simulink model "vbyfcontrolim_interrupt"  (R2016a)
settings: Solver=ode4  StartTime=0.0  StopTime=20  FixedStep=Ts  RelTol=1e-3
values from neighbouring files (symbols this model uses):
  Cdc = 100e-6    (= 0.0001)    [control_simulation_parameters.m]    (also in pmsm_vbyf_sim_parameters.m = 1.5e-05; vbyfcontrolim_sim.m)
  deltad = delta*180/pi    [control_simulation_parameters.m]    (also in pmsm_vbyf_sim_parameters.m)
  Ef = 155    [control_simulation_parameters.m]    (also in pmsm_vbyf_sim_parameters.m = 80)
  fout = 50    [control_simulation_parameters.m]    (also in pmsm_vbyf_sim_parameters.m = 100; vbyfcontrolim_sim.m)
  frated = 50    [vbyfcontrolim_sim.m]
  fsw = 10e3    (= 10000)    [control_simulation_parameters.m]    (also in pmsm_vbyf_sim_parameters.m; vbyfcontrolim_sim.m)
  Ls = 13.8e-3    (= 0.0138)    [control_simulation_parameters.m]
  phase = [0 90 0 90]    [control_simulation_parameters.m]    (also in pmsm_vbyf_sim_parameters.m = [0])
  Rin = 10    [control_simulation_parameters.m]    (also in pmsm_vbyf_sim_parameters.m = 1; vbyfcontrolim_sim.m = 1e-06)
  Ripth = 0.08    [control_simulation_parameters.m]    (also in pmsm_vbyf_sim_parameters.m; vbyfcontrolim_sim.m)
  Rs = 1e-3    (= 0.001)    [control_simulation_parameters.m]
  Tload = 30    [pmsm_vbyf_sim_parameters.m]    (also in vbyfcontrolim_sim.m = 10)
  Trated = Prated/wrated    (= 26.7113191203)    [vbyfcontrolim_sim.m]
  Ts = 100e-9    (= 1e-07)    [control_simulation_parameters.m]    (also in pmsm_vbyf_sim_parameters.m = 1e-06; vbyfcontrolim_sim.m = 1e-06)
  VbyfFreqSteps = 2    [vbyfcontrolim_sim.m]
  VbyfStepTime = 0.2    [vbyfcontrolim_sim.m]
  Vdc = 300    [control_simulation_parameters.m]    (also in pmsm_vbyf_sim_parameters.m = 270; vbyfcontrolim_sim.m = 750)
  Vin = Vdc + Rin*(Pout/Vdc)    (= 366.666666667)    [control_simulation_parameters.m]    (also in pmsm_vbyf_sim_parameters.m = 276.981317008; vbyfcontrolim_sim.m = 750)
  Vrated = Vllrated/sqrt(3)    [vbyfcontrolim_sim.m]
undefined symbols (not defined in the file or in its folder): Initial_freq, Lload, Rload, start_time, start_time_deceleration
libraries: powerlib x25, powerlib_meascontrol x14, simulink x4, dspsigops x2
settings Model: SimulationMode=accelerator  Creator=ugurm  LastModifiedBy=mesutto
settings DataIOCC: LimitDataPoints=on  SaveFormat=Array
settings DebuggingCC: UnderspecifiedInitializationDetection=Classic  MergeDetectMultiDrivingBlocksExec=none  SolverPrmCheckMsg=warning  StateNameClashWarn=warning
settings HardwareCC: ProdBitPerPointer=32  ProdLargestAtomicFloat=None  ProdIntDivRoundTo=Undefined  ProdEndianess=Unspecified  ProdWordSize=32  ProdHWDeviceType=32-bit Generic
settings ModelReferenceCC: PropagateSignalLabelsOutOfModel=off
settings ConfigComp: CovModelRefEnable=Off

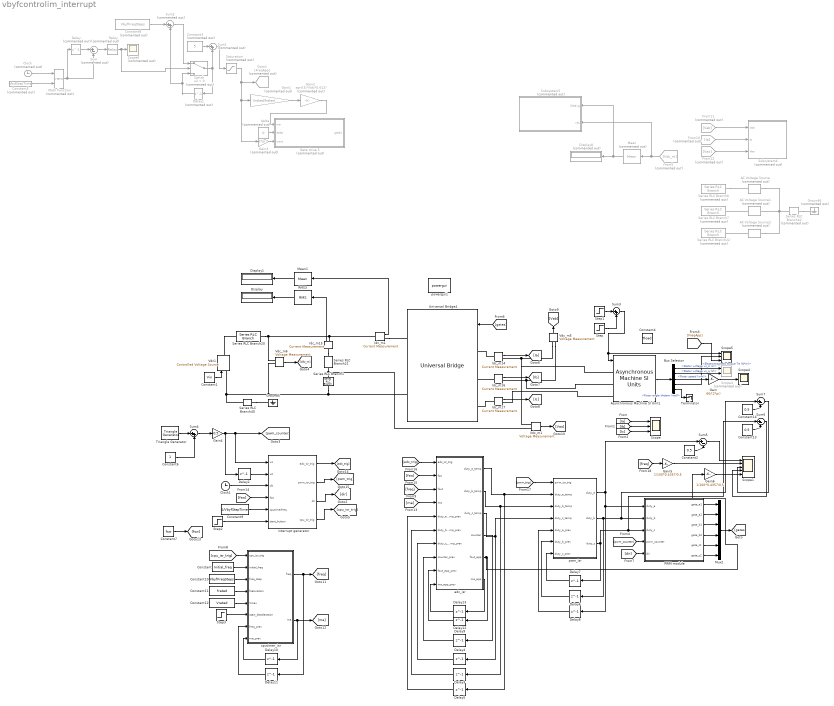
== system vbyfcontrolim_interrupt ==
  AC Voltage Source : powerlib/Electrical Sources/AC Voltage Source  Commented=on  Amplitude=Ef*sqrt(2)  Phase=0  Frequency=fout  SampleTime=0  Measurements=None  BusType=swing  Pref=10e3  Qref=0  Qmin=-inf  Qmax=+inf
  AC Voltage Source1 : powerlib/Electrical Sources/AC Voltage Source  Commented=on  Amplitude=Ef*sqrt(2)  Phase=-120  Frequency=fout  SampleTime=0  Measurements=None  BusType=swing  Pref=10e3  Qref=0  Qmin=-inf  Qmax=+inf
  AC Voltage Source2 : powerlib/Electrical Sources/AC Voltage Source  Commented=on  Amplitude=Ef*sqrt(2)  Phase=-240  Frequency=fout  SampleTime=0  Measurements=None  BusType=swing  Pref=10e3  Qref=0  Qmin=-inf  Qmax=+inf
  Asynchronous Machine SI Units : powerlib/Machines/Asynchronous Machine SI Units  RotorType=Squirrel-cage  PresetModel=No  MechanicalLoad=Torque Tm  ShowDetailedParameters=on  ReferenceFrame=Synchronous  Units=SI  MeasurementBus=off  NominalParameters=[4000 400 50]  Stator=[1.405 0.005839]  Rotor=[1.395 0.005839]  Cage1=[0.4155 0.002066]  Cage2=[0.4168 0.0003495]  Lm=0.1722  Mechanical=[0.0131 0.002985 2]  PolePairs=2  InitialConditions=[1 0 0 0 0 0 0 0]  SimulateSaturation=off  Saturation=[14.03593122, 27.81365428, 53.79336849, 72.68890987, 97.98006896, 148.6815601, 215.7428561, 302.9841135, 428.7778367 ; 230, 322, 414, 460, 506, 552, 598, 644, 690]  LoadFlowParameters=1492000  TsPowergui=0  TsBlock=-1  IterativeModel=Trapezoidal non iterative  IterativeDiscreteModel=Trapezoidal non iterative  Pmec=1.492e+006
  Bus Selector : BusSelector  OutputSignals=Stator measurements.Stator voltage vs_d (V),Stator measurements.Stator voltage vs_q (V),Mechanical.Rotor speed (wm),Mechanical.Electromagnetic torque Te (N*m),Mechanical.Rotor angle thetam (rad)
  Clock : Clock  Commented=on
  Clock1 : Clock
  Constant : Constant  Value=Initial_freq
  Constant1 : Constant  Value=Vin
  Constant10 : Constant  Value=VbyfFreqSteps
  Constant11 : Constant  Value=frated
  Constant12 : Constant  Value=Vrated
  Constant13 : Constant  Value=0.5
  Constant14 : Constant  Value=0.5
  Constant2 : Constant  Value=0.5
  Constant3 : Constant  Commented=on  Value=5
  Constant4 : Constant  Value=Tload
  Constant5 : Constant  Commented=on  Value=VbyfStepTime
  Constant6 : Constant
  Constant7 : Constant  Value=fsw
  Constant8 : Constant  Commented=on  Value=VbyfFreqSteps
  Constant9 : Constant  Value=1/VbyfStepTime
  Delay : Delay  Commented=on  DelayLength=1
  Delay1 : Delay  Commented=on  DelayLength=1
  Delay{2..13} (12 alike) : Delay  DelayLength=1
  Display : Display
  Display1 : Display
  Display8 : Display  Commented=on
  From10 : From  Commented=on  GotoTag=Ia
  From11 : From  Commented=on  GotoTag=Vab
  From12 : From  Commented=on  GotoTag=Vao
  From5 : From  Commented=on  GotoTag=Vdc_m
  Gain : Gain  Gain=60/(2*pi)
  Gain1 : Gain  Commented=on  Gain=Vrated/frated
  Gain2 : Gain  Commented=on  Gain=sqrt(3)/(Vdc*0.612)
  Gain3 : Gain  Commented=on  Gain=2*pi
  Gain4 : Gain  Gain=0.5
  Gain5 : Gain  Gain=1/100*0.4357/0.5
  Gain6 : Gain  Gain=1/100*0.4357/0.5
  Gate drive 5 : Subsystem  Commented=on
  Goto1 : Goto  Commented=on  GotoTag=FreqApp
  Ground5 : powerlib/Elements/Ground  LConnTagsString=a
  Ground6 : powerlib/Elements/Ground  Commented=on  LConnTagsString=a
  Idc_m{1,14..17} (5 alike) : powerlib/Measurements/Current Measurement  PhasorSimulation=off  OutputType=Complex  PSBequivalent=0
  Math Function : Math  Commented=on  Operator=rem  SaturateOnIntegerOverflow=on
  Mean : powerlib_meascontrol/Measurements/Mean  Commented=on  Freq=fout  Vinit=0  Ts=0
  Mean1 : powerlib_meascontrol/Measurements/Mean  Freq=fout  Vinit=0  Ts=0
  Mux2 : Mux  Inputs=6
  PWM module : MATLAB Function  TreatAsAtomicUnit=on
  RMS3 : powerlib_meascontrol/Measurements/RMS  TrueRMS=on  Freq=fout  RMSInit=0  Ts=0
  Relay : Relay  Commented=on
  Saturation : Saturate  Commented=on  UpperLimit=frated  LowerLimit=0
  Scope : Scope  NumInputPorts=3
  Scope1 : Scope  NumInputPorts=5
  Scope3 : Scope  Commented=on  NumInputPorts=2
  Scope4 : Scope
  Scope5 : Scope  NumInputPorts=3
  Scope6 : Scope  Commented=on
  Series RLC Branch1 : powerlib/Elements/Series RLC Branch  LConnTagsString=__new0  RConnTagsString=__new0  BranchType=C  Resistance=Rload  Inductance=Lload  SetiL0=off  InitialCurrent=0  Capacitance=Cdc*2  Setx0=off  InitialVoltage=0  Measurements=None
  Series RLC Branch20 : powerlib/Elements/Series RLC Branch  LConnTagsString=__new0  RConnTagsString=__new0  BranchType=R  Resistance=Rin  Inductance=Lload  SetiL0=off  InitialCurrent=0  Capacitance=1e-6  Setx0=off  InitialVoltage=0  Measurements=None
  Series RLC Branch21 : powerlib/Elements/Series RLC Branch  LConnTagsString=__new0  RConnTagsString=__new0  BranchType=C  Resistance=Rload  Inductance=Lload  SetiL0=off  InitialCurrent=0  Capacitance=Cdc*2  Setx0=off  InitialVoltage=0  Measurements=None
  Series RLC Branch22 : powerlib/Elements/Series RLC Branch  Commented=on  LConnTagsString=__new0  RConnTagsString=__new0  BranchType=RL  Resistance=Rs  Inductance=Ls  SetiL0=off  InitialCurrent=0  Capacitance=1e-6  Setx0=off  InitialVoltage=0  Measurements=None
  Series RLC Branch40 : powerlib/Elements/Series RLC Branch  LConnTagsString=__new0  RConnTagsString=__new0  BranchType=R  Resistance=1e12  Inductance=Lload  SetiL0=off  InitialCurrent=0  Capacitance=1e-6  Setx0=off  InitialVoltage=0  Measurements=None
  Series RLC Branch42 : powerlib/Elements/Series RLC Branch  Commented=on  LConnTagsString=__new0  RConnTagsString=__new0  BranchType=R  Resistance=1e12  Inductance=Lload  SetiL0=off  InitialCurrent=0  Capacitance=1e-6  Setx0=off  InitialVoltage=0  Measurements=None
  Series RLC Branch6 : powerlib/Elements/Series RLC Branch  Commented=on  LConnTagsString=__new0  RConnTagsString=__new0  BranchType=RL  Resistance=Rs  Inductance=Ls  SetiL0=off  InitialCurrent=0  Capacitance=1e-6  Setx0=off  InitialVoltage=0  Measurements=None
  Series RLC Branch7 : powerlib/Elements/Series RLC Branch  Commented=on  LConnTagsString=__new0  RConnTagsString=__new0  BranchType=RL  Resistance=Rs  Inductance=Ls  SetiL0=off  InitialCurrent=0  Capacitance=1e-6  Setx0=off  InitialVoltage=0  Measurements=None
  Step : Step  Time=2  After=Tload  SampleTime=0
  Step1 : Step  Time=6  After=Trated-Tload  SampleTime=0
  Step2 : Step  Time=start_time  SampleTime=0
  Step3 : Step  Time=start_time_deceleration  SampleTime=0
  Subsystem4 : Subsystem  Commented=on
  Subsystem5 : Subsystem  Commented=on
  Sum : Sum  Commented=on  Inputs=|+-
  Sum1 : Sum  Commented=on  Inputs=|++
  Sum2 : Sum  Commented=on  Inputs=|++
  Sum3 : Sum  Inputs=|++
  Sum4 : Sum  Inputs=|++
  Sum5 : Sum  Inputs=|+-
  Sum6 : Sum  Inputs=|+-
  Sum7 : Sum  Inputs=|+-
  Switch : Switch  Commented=on  Criteria=u2 > Threshold
  Terminator : Terminator
  Triangle Generator : powerlib_meascontrol/Pulse & Signal Generators/Triangle Generator  Freq=fsw  Phase=0  Ts=0
  Universal Bridge4 : powerlib/Power Electronics/Universal Bridge  Arms=3  SnubberResistance=1e5  SnubberCapacitance=inf  Device=IGBT / Diodes  Ron=1e-6  Lon=0  ForwardVoltages="[  0  0  ]"  ForwardVoltage=0  GTOparameters=[ 10e-6 , 20e-6 ]  IGBTparameters=[0,0]  Measurements=None  Measurements_2=None  converterType=Rectifier
  Vdc1 : powerlib/Electrical Sources/Controlled Voltage Source  Initialize=off  Source_Type=DC  Amplitude=200  Phase=0  Frequency=0  Measurements=None
  Vdc_m1 : powerlib/Measurements/Voltage Measurement  PhasorSimulation=off  OutputType=Complex  PSBequivalent=0
  Vdc_m5 : powerlib/Measurements/Voltage Measurement  PhasorSimulation=off  OutputType=Complex  PSBequivalent=0
  Vdc_m6 : powerlib/Measurements/Voltage Measurement  PhasorSimulation=off  OutputType=Complex  PSBequivalent=0
  adc_isr : MATLAB Function  TreatAsAtomicUnit=on
  cputimer_isr : MATLAB Function  TreatAsAtomicUnit=on
  delta : Constant  Commented=on  Value=0
  interrupt generator : MATLAB Function  TreatAsAtomicUnit=on
  powergui1 : powerlib/powergui  Priority=1  SimulationMode=Discrete  SolverType=Tustin  SampleTime=Ts  frequency=60  SPID=off  DisableSnubberDevices=off  DisableRonSwitches=off  DisableVfSwitches=off  SwTol=0  DisplayEquations=off  Interpol=off  ExternalGateDelay=off  methode=off  Ts=0  FunctionMessages=off  echomessages=off  HookPort=off  EnableUseOfTLC=off  x0status=blocks  frequencyindice=0  Pbase=100e6  ErrMax=1e-4  Iterations=50  UnitsV=kV  UnitsW=MW  buscounter=0  RestoreLinks=warning  ResistiveCurrentMeasurement=off  Frange=[0:2:500]  Ylog=off  Xlog=on  ShowGrid=off  save=off  variable=ZData  structure=Vdc  ZoomFFT=off  StartTime=0.04  cycles=5  DisplayStyle=5  fundamental=50  FreqAxis=off  MaxFrequency=30000  frequencyindicesteady=1  RmsSteady=1  display=off
  pwm_isr : MATLAB Function  TreatAsAtomicUnit=on
  wires:
  Constant1/1 -> Vdc1/1
  Idc_m15/1 -> RMS3/1
  Vdc_m6/1 -> [Vdc_m]
  RMS3/1 -> Display/1
  Mean/1 -> Subsystem5/1(Vdcavg), Display8/1
  Idc_m1/1 -> Mean1/1
  Mean1/1 -> Display1/1
  Idc_m14/1 -> [Ia]
  From5/1 -> Subsystem5/2(vdc), Mean/1
  From10/1 -> Subsystem4/2(Ia)
  Idc_m16/1 -> [Ib]
  Idc_m17/1 -> [Ic]
  From11/1 -> Subsystem4/1(Vab)
  From12/1 -> Subsystem4/3(Vao)
  Vdc_m5/1 -> [Vab]
  Vdc_m1/1 -> [Vao]
  [Ia] -> Scope/1
  [Ic] -> Scope/3
  [Ib] -> Scope/2
  delta/1 -> Gate drive 5/2(delta)
  Asynchronous Machine SI Units/1 -> Bus Selector/1
  Bus Selector/1 -> Scope3/1  "<Stator voltage vs_d (V)>"
  Bus Selector/2 -> Scope3/2  "<Stator voltage vs_q (V)>"
  Bus Selector/3 -> Gain/1  "<Rotor speed (wm)>"
  Bus Selector/4 -> Scope5/2  "<Electromagnetic torque Te (N*m)>"
  Bus Selector/5 -> Terminator/1  "<Rotor angle thetam (rad)>"
  Gain/1 -> Scope4/1
  Clock/1 -> Math Function/1
  Constant5/1 -> Math Function/2
  Math Function/1 -> Sum/2, Delay/1
  Delay/1 -> Sum/1
  Sum/1 -> Relay/1
  Relay/1 -> Switch/2, Scope6/1
  Sum2/1 -> Switch/1
  Constant8/1 -> Sum2/1
  Delay1/1 -> Switch/3, Sum2/2
  Switch/1 -> Sum1/2, Delay1/1
  Gain1/1 -> Gain2/1
  Gain2/1 -> Gate drive 5/1(ma)
  Gain3/1 -> Gate drive 5/3(wout)
  Saturation/1 -> Goto1/1, Gain3/1, Gain1/1
  Step/1 -> Sum3/2
  [FreqApp] -> Scope5/3
  Constant3/1 -> Sum1/1
  Sum1/1 -> Saturation/1
  Step1/1 -> Sum3/1
  Sum3/1 -> Asynchronous Machine SI Units/1, Scope5/1
  Triangle Generator/1 -> Sum4/1
  Constant6/1 -> Sum4/2
  Sum4/1 -> Gain4/1
  Gain4/1 -> [pwm_counter], interrupt generator/1(u1), Delay2/1
  Delay2/1 -> interrupt generator/2(u2)
  Clock1/1 -> interrupt generator/3(clk)
  adc_isr/1(duty_a_temp) -> Delay5/1, pwm_isr/2(duty_a_temp)
  adc_isr/2(duty_b_temp) -> Delay3/1, pwm_isr/3(duty_b_temp)
  adc_isr/3(duty_c_temp) -> pwm_isr/4(duty_c_temp), Delay4/1
  [pwm_counter] -> PWM module/4(pwm_counter)
  PWM module/6(gate_c2) -> Mux2/6
  PWM module/4(gate_b2) -> Mux2/4
  PWM module/5(gate_c1) -> Mux2/5
  PWM module/3(gate_b1) -> Mux2/3
  PWM module/2(gate_a2) -> Mux2/2
  PWM module/1(gate_a1) -> Mux2/1
  [gates] -> Universal Bridge4/1
  Mux2/1 -> [gates]
  [dir] -> PWM module/5(dir)
  interrupt generator/3(dir) -> [dir]
  Delay5/1 -> adc_isr/5(duty_a_temp_prev)
  Delay3/1 -> adc_isr/6(duty_b_temp_prev)
  Delay4/1 -> adc_isr/7(duty_c_temp_prev)
  Delay7/1 -> pwm_isr/7(duty_c_prev)
  Delay6/1 -> pwm_isr/6(duty_b_prev)
  Delay8/1 -> pwm_isr/5(duty_a_prev)
  pwm_isr/3(duty_c) -> Delay7/1, Sum6/1, PWM module/3(duty_c)
  pwm_isr/1(duty_a) -> Sum5/1, PWM module/1(duty_a), Delay8/1
  [fsw] -> interrupt generator/4(fsw)
  [freq] -> adc_isr/3(fout)
  Delay9/1 -> adc_isr/8(counter_prev)
  Constant9/1 -> interrupt generator/5(cputimerfreq)
  Constant/1 -> cputimer_isr/2(initial_freq)
  interrupt generator/4(cpu_isr_trig) -> [cpu_isr_trig]
  [cpu_isr_trig] -> cputimer_isr/1(cpu_isr_trig)
  Constant10/1 -> cputimer_isr/3(freq_step)
  Constant11/1 -> cputimer_isr/4(fsaturation)
  Constant12/1 -> cputimer_isr/5(Vmax)
  cputimer_isr/2(ma) -> [ma], Delay10/1
  Delay10/1 -> cputimer_isr/8(ma_prev)
  cputimer_isr/1(freq) -> [freq], Delay11/1
  Delay11/1 -> cputimer_isr/7(freq_prev)
  [ma] -> adc_isr/4(ma)
  Constant7/1 -> [fsw]
  [fsw] -> adc_isr/2(fsw)
  interrupt generator/1(adc_isr_trig) -> [adc_trig]
  [adc_trig] -> adc_isr/1(adc_isr_trig)
  interrupt generator/2(pwm_isr_trig) -> [pwm_trig]
  [pwm_trig] -> pwm_isr/1(pwm_isr_trig)
  adc_isr/5(fout_app) -> Gain6/1, Delay12/1
  adc_isr/6(ma_app) -> Delay13/1
  Delay13/1 -> adc_isr/10(ma_app_prev)
  Delay12/1 -> adc_isr/9(fout_app_prev)
  Gain5/1 -> Scope1/2
  [freq] -> Gain5/1
  adc_isr/4(counter) -> Delay9/1
  Constant2/1 -> Sum5/2
  Sum5/1 -> Scope1/1
  Constant13/1 -> Sum6/2
  Constant14/1 -> Sum7/2
  pwm_isr/2(duty_b) -> Sum7/1, PWM module/2(duty_b), Delay6/1
  Sum7/1 -> Scope1/3
  Sum6/1 -> Scope1/4
  Gain6/1 -> Scope1/5
  Step2/1 -> interrupt generator/6(start_button)
  Step3/1 -> cputimer_isr/6(start_deceleration)
  connections:
  Vdc_m5/LConn1 -- Asynchronous Machine SI Units/LConn1 -- Vdc_m1/LConn1 -- Idc_m14/RConn1
  Universal Bridge4/RConn2 -- Vdc_m6/LConn2 -- Vdc1/LConn1 -- Series RLC Branch40/LConn1 -- Series RLC Branch1/RConn1
  Series RLC Branch42/RConn1 -- Ground6/LConn1
  Series RLC Branch40/RConn1 -- Ground5/LConn1
  Idc_m14/LConn1 -- Universal Bridge4/LConn1
  Idc_m15/LConn1 -- Series RLC Branch21/LConn1
  Vdc1/RConn1 -- Series RLC Branch20/LConn1
  Series RLC Branch6/RConn1 -- AC Voltage Source/RConn1
  AC Voltage Source1/RConn1 -- Series RLC Branch7/RConn1
  AC Voltage Source2/RConn1 -- Series RLC Branch22/RConn1
  Series RLC Branch42/LConn1 -- AC Voltage Source/LConn1 -- AC Voltage Source2/LConn1 -- AC Voltage Source1/LConn1
  Idc_m16/LConn1 -- Universal Bridge4/LConn2
  Idc_m17/LConn1 -- Universal Bridge4/LConn3
  Vdc_m5/LConn2 -- Asynchronous Machine SI Units/LConn2 -- Idc_m16/RConn1
  Idc_m1/RConn1 -- Universal Bridge4/RConn1
  Idc_m1/LConn1 -- Series RLC Branch20/RConn1 -- Vdc_m6/LConn1 -- Idc_m15/RConn1
  Series RLC Branch1/LConn1 -- Vdc_m1/LConn2 -- Series RLC Branch21/RConn1
  Asynchronous Machine SI Units/LConn3 -- Idc_m17/RConn1

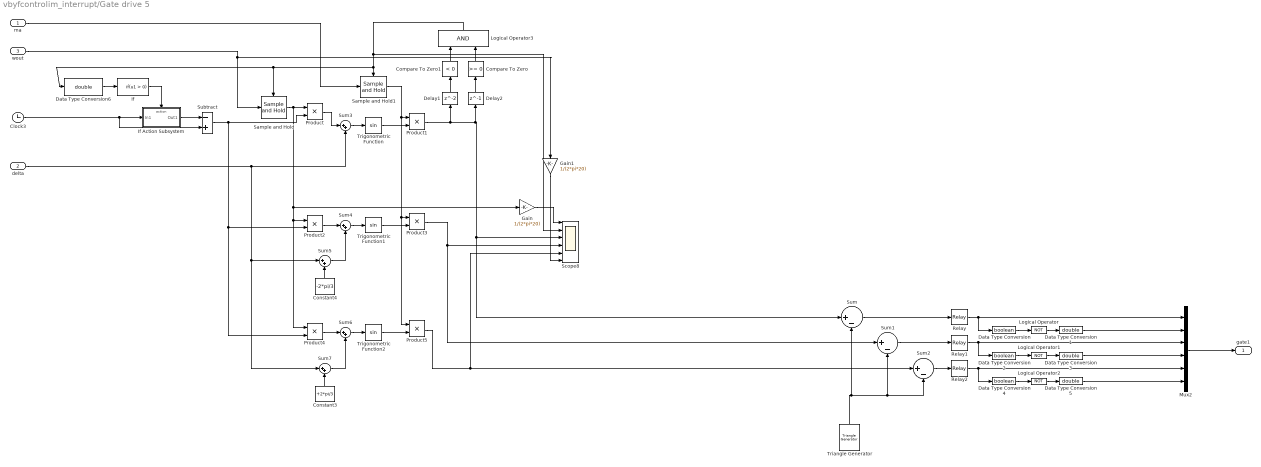
== system vbyfcontrolim_interrupt/Gate drive 5 ==
  ma : Inport
  delta : Inport  Port=2
  wout : Inport  Port=3
  Clock3 : Clock
  Compare To Zero : simulink/Logic and Bit Operations/Compare To Zero  relop=>=  OutDataTypeStr=boolean
  Compare To Zero1 : simulink/Logic and Bit Operations/Compare To Zero  relop=<  OutDataTypeStr=boolean
  Constant3 : Constant  Value=+2*pi/3
  Constant4 : Constant  Value=-2*pi/3
  Data Type Conversion : DataTypeConversion  OutDataTypeStr=boolean
  Data Type Conversion{1,3,5..6} (4 alike) : DataTypeConversion  OutDataTypeStr=double
  Data Type Conversion2 : DataTypeConversion  OutDataTypeStr=boolean
  Data Type Conversion4 : DataTypeConversion  OutDataTypeStr=boolean
  Delay1 : Delay
  Delay2 : Delay  DelayLength=1
  Gain : Gain  Gain=1/(2*pi*20)
  Gain1 : Gain  Gain=1/(2*pi*20)
  If : If  ShowElse=off
  If Action Subsystem : Subsystem  TreatAsAtomicUnit=on
  Logical Operator : Logic  Operator=NOT  AllPortsSameDT=off  OutDataTypeStr=boolean
  Logical Operator1 : Logic  Operator=NOT  AllPortsSameDT=off  OutDataTypeStr=boolean
  Logical Operator2 : Logic  Operator=NOT  AllPortsSameDT=off  OutDataTypeStr=boolean
  Logical Operator3 : Logic  AllPortsSameDT=off  OutDataTypeStr=boolean
  Mux2 : Mux  Inputs=6
  Product{,1..5} (6 alike) : Product
  Relay : Relay
  Relay1 : Relay
  Relay2 : Relay
  Sample and Hold : dspsigops/Sample and Hold  trig=Rising edge  initCond=5*2*pi  latchinput=off
  Sample and Hold1 : dspsigops/Sample and Hold  trig=Rising edge  initCond=5/frated*Vrated*sqrt(3)/(Vdc*0.612)  latchinput=on
  Scope8 : Scope  NumInputPorts=6
  Subtract : Sum  Inputs=-+
  Sum : Sum  Inputs=|+-
  Sum1 : Sum  Inputs=|+-
  Sum2 : Sum  Inputs=|+-
  Sum{3..7} (5 alike) : Sum  Inputs=|++
  Triangle Generator : powerlib_meascontrol/Pulse & Signal Generators/Triangle Generator  Freq=fsw  Phase=phase(1)  Ts=Ts
  Trigonometric Function : Trigonometry
  Trigonometric Function1 : Trigonometry
  Trigonometric Function2 : Trigonometry
  gate1 : Outport
  wires:
  Triangle Generator/1 -> Sum1/2, Sum2/2, Sum/2
  Product3/1 -> Scope8/4, Sum1/1
  Product5/1 -> Scope8/5, Sum2/1
  Sum/1 -> Relay/1
  Sum1/1 -> Relay1/1
  Sum2/1 -> Relay2/1
  Data Type Conversion/1 -> Logical Operator/1
  Relay/1 -> Data Type Conversion/1, Mux2/1
  Logical Operator/1 -> Data Type Conversion1/1
  Data Type Conversion1/1 -> Mux2/2
  Data Type Conversion2/1 -> Logical Operator1/1
  Relay1/1 -> Data Type Conversion2/1, Mux2/3
  Logical Operator1/1 -> Data Type Conversion3/1
  Data Type Conversion3/1 -> Mux2/4
  Data Type Conversion4/1 -> Logical Operator2/1
  Relay2/1 -> Data Type Conversion4/1, Mux2/5
  Logical Operator2/1 -> Data Type Conversion5/1
  Data Type Conversion5/1 -> Mux2/6
  Mux2/1 -> gate1/1
  Trigonometric Function/1 -> Product1/2
  Sum3/1 -> Trigonometric Function/1
  Product/1 -> Sum3/1
  Trigonometric Function1/1 -> Product3/2
  Sum4/1 -> Trigonometric Function1/1
  Product2/1 -> Sum4/1
  Sum5/1 -> Sum4/2
  Constant4/1 -> Sum5/2
  wout/1 -> Gain1/1, Sample and Hold/1
  ma/1 -> Sample and Hold1/1
  delta/1 -> Sum3/2, Sum7/1, Sum5/1
  Trigonometric Function2/1 -> Product5/2
  Sum6/1 -> Trigonometric Function2/1
  Product4/1 -> Sum6/1
  Sum7/1 -> Sum6/2
  Constant3/1 -> Sum7/2
  Sample and Hold/1 -> Gain/1, Product2/1, Product4/1, Product/1
  Product1/1 -> Delay1/1, Scope8/3, Sum/1, Delay2/1
  Delay1/1 -> Compare To Zero1/1
  Compare To Zero/1 -> Logical Operator3/2
  Compare To Zero1/1 -> Logical Operator3/1
  Logical Operator3/1 -> Data Type Conversion6/1, Sample and Hold/Trigger, Sample and Hold1/Trigger, Scope8/2
  Delay2/1 -> Compare To Zero/1
  Subtract/1 -> Product4/2, Product2/2, Product/2
  If/1 -> If Action Subsystem/Action
  Clock3/1 -> Subtract/2, If Action Subsystem/1(In1)
  If Action Subsystem/1(Out1) -> Subtract/1
  Data Type Conversion6/1 -> If/1
  Sample and Hold1/1 -> Product3/1, Product5/1, Product1/1
  Gain/1 -> Scope8/1
  Gain1/1 -> Scope8/6

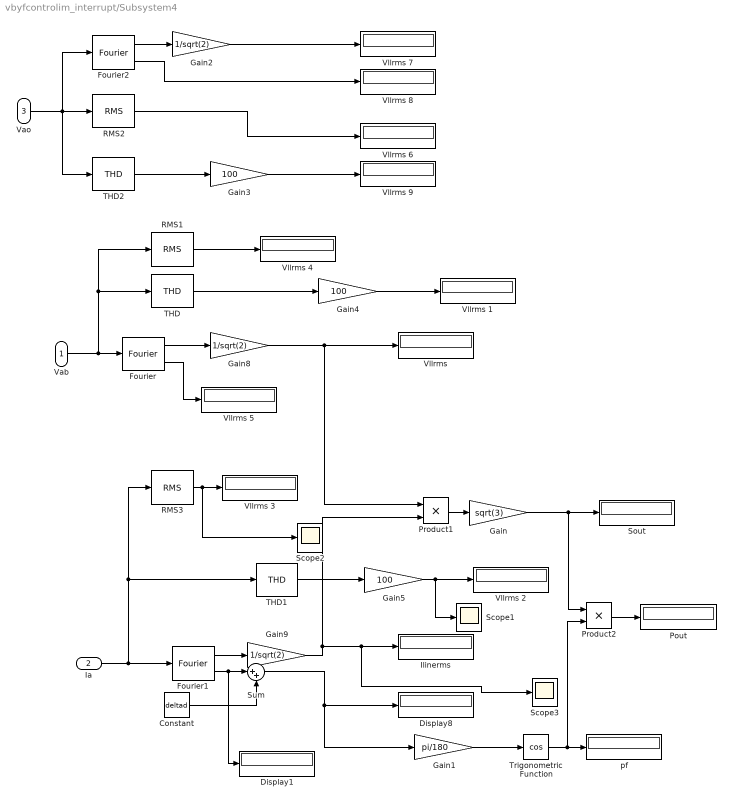
== system vbyfcontrolim_interrupt/Subsystem4 ==
  Vab : Inport
  Ia : Inport  Port=2
  Vao : Inport  Port=3
  Constant : Constant  Value=deltad
  Display1 : Display
  Display8 : Display
  Fourier : powerlib_meascontrol/Measurements/Fourier  Freq=fout  n=1  InInit=[0, 0]  Ts=Ts
  Fourier1 : powerlib_meascontrol/Measurements/Fourier  Freq=fout  n=1  InInit=[0, 0]  Ts=Ts
  Fourier2 : powerlib_meascontrol/Measurements/Fourier  Freq=fout  n=1  InInit=[0, 0]  Ts=Ts
  Gain : Gain  Gain=sqrt(3)
  Gain1 : Gain  Gain=pi/180
  Gain2 : Gain  Gain=1/sqrt(2)
  Gain3 : Gain  Gain=100
  Gain4 : Gain  Gain=100
  Gain5 : Gain  Gain=100
  Gain8 : Gain  Gain=1/sqrt(2)
  Gain9 : Gain  Gain=1/sqrt(2)
  "Ilinerms " : Display
  Pout : Display
  Product1 : Product
  Product2 : Product
  RMS1 : powerlib_meascontrol/Measurements/RMS  TrueRMS=on  Freq=fout  RMSInit=0  Ts=0
  RMS2 : powerlib_meascontrol/Measurements/RMS  TrueRMS=on  Freq=fout  RMSInit=0  Ts=0
  RMS3 : powerlib_meascontrol/Measurements/RMS  TrueRMS=on  Freq=fout  RMSInit=0  Ts=0
  Scope1 : Scope
  Scope2 : Scope
  Scope3 : Scope
  Sout : Display
      settings: Format=short_e
  Sum : Sum  Inputs=|++
  THD : powerlib_meascontrol/Measurements/THD  Freq=fout  Ts=0
  THD1 : powerlib_meascontrol/Measurements/THD  Freq=fout  Ts=0
  THD2 : powerlib_meascontrol/Measurements/THD  Freq=fout  Ts=0
  Trigonometric Function : Trigonometry  Operator=cos
  Vllrms {,1..9} (10 alike) : Display
  pf : Display
  wires:
  Gain8/1 -> Product1/1, "Vllrms "/1
  Gain9/1 -> Scope3/1, "Ilinerms "/1, Product1/2
  Ia/1 -> RMS3/1, THD1/1, Fourier1/1
  Fourier1/1 -> Gain9/1
  Vab/1 -> RMS1/1, THD/1, Fourier/1
  Fourier/1 -> Gain8/1
  Product1/1 -> Gain/1
  Gain/1 -> Product2/1, Sout/1
  Sum/1 -> Gain1/1, Display8/1
  Trigonometric Function/1 -> Product2/2, pf/1
  Gain1/1 -> Trigonometric Function/1
  Product2/1 -> Pout/1
  Fourier/2 -> Vllrms 5/1
  THD/1 -> Gain4/1
  THD1/1 -> Gain5/1
  Constant/1 -> Sum/2
  RMS3/1 -> Scope2/1, Vllrms 3/1
  RMS1/1 -> Vllrms 4/1
  Fourier1/2 -> Display1/1, Sum/1
  Vao/1 -> THD2/1, Fourier2/1, RMS2/1
  RMS2/1 -> Vllrms 6/1
  Fourier2/1 -> Gain2/1
  Fourier2/2 -> Vllrms 8/1
  Gain2/1 -> Vllrms 7/1
  THD2/1 -> Gain3/1
  Gain3/1 -> Vllrms 9/1
  Gain4/1 -> Vllrms 1/1
  Gain5/1 -> Scope1/1, Vllrms 2/1

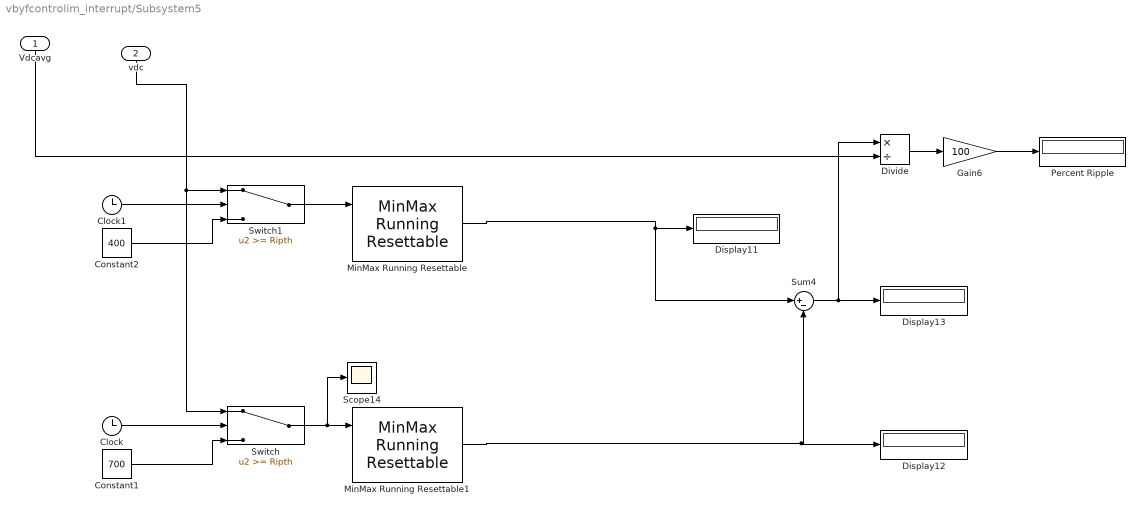
== system vbyfcontrolim_interrupt/Subsystem5 ==
  Vdcavg : Inport
  vdc : Inport  Port=2
  Clock : Clock
  Clock1 : Clock
  Constant1 : Constant  Value=700  SampleTime=Ts
  Constant2 : Constant  Value=400  SampleTime=Ts
  Display11 : Display
  Display12 : Display
  Display13 : Display
  Divide : Product  Inputs=*/
  Gain6 : Gain  Gain=100
  MinMax Running Resettable : simulink/Math Operations/MinMax Running Resettable  Function=max  vinit=0.0
  MinMax Running Resettable1 : simulink/Math Operations/MinMax Running Resettable  Function=min  vinit=700
  Percent Ripple : Display
  Scope14 : Scope
  Sum4 : Sum  Inputs=|+-
  Switch : Switch  Threshold=Ripth
  Switch1 : Switch  Threshold=Ripth
  wires:
  MinMax Running Resettable/1 -> Display11/1, Sum4/1
  Clock/1 -> Switch/2
  Gain6/1 -> Percent Ripple/1
  Constant1/1 -> Switch/3
  MinMax Running Resettable1/1 -> Display12/1, Sum4/2
  Switch/1 -> Scope14/1, MinMax Running Resettable1/1
  Sum4/1 -> Divide/1, Display13/1
  Divide/1 -> Gain6/1
  Vdcavg/1 -> Divide/2
  vdc/1 -> Switch1/1, Switch/1
  Switch1/1 -> MinMax Running Resettable/1
  Clock1/1 -> Switch1/2
  Constant2/1 -> Switch1/3

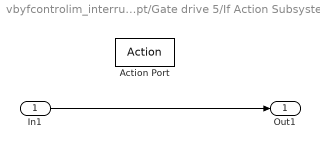
== system vbyfcontrolim_interrupt/Gate drive 5/If Action Subsystem ==
  In1 : Inport
  Action Port : ActionPort  ActionType=then
  Out1 : Outport
  wires:
  In1/1 -> Out1/1

== matlab function vbyfcontrolim_interrupt/adc_isr ==
  data: adc_isr_trig input; fsw input; fout input; ma input; duty_a_temp_prev input; duty_b_temp_prev input; duty_c_temp_prev input; counter_prev input; duty_a_temp output; duty_b_temp output; duty_c_temp output; counter output; fout_app_prev input; ma_app_prev input; fout_app output; ma_app output
function [duty_a_temp,duty_b_temp,duty_c_temp,counter,fout_app,ma_app] = fcn(adc_isr_trig,...
    fsw,fout,ma,duty_a_temp_prev,duty_b_temp_prev,duty_c_temp_prev,counter_prev,fout_app_prev,ma_app_prev)

if (adc_isr_trig == 1) % interrupt on zero event
    counter = counter_prev+1;
    fout_app = fout_app_prev;
    if(counter > (fsw/fout_app)-1)
        counter = 0;
        fout_app = fout;
        ma_app = ma;
    else
        fout_app = fout_app_prev;
        ma_app = ma_app_prev;
    end
    duty_a_temp = (ma_app*sin(2*pi*fout_app*counter/fsw)+1)/2;
    duty_b_temp = (ma_app*sin(2*pi*fout_app*counter/fsw-2*pi/3)+1)/2;
    duty_c_temp = (ma_app*sin(2*pi*fout_app*counter/fsw+2*pi/3)+1)/2;
else
    duty_a_temp = duty_a_temp_prev;
    duty_b_temp = duty_b_temp_prev;
    duty_c_temp = duty_c_temp_prev;
    counter = counter_prev;
    %fout_app = fout_app_prev;
    %ma_app = ma_app_prev;
    if (fout_app_prev == 0)
       ma_app = ma;
       fout_app = fout;
    else
        ma_app = ma_app_prev;
        fout_app = fout_app_prev;
    end
end;

== matlab function vbyfcontrolim_interrupt/pwm_isr ==
  data: duty_a output; pwm_isr_trig input; duty_a_temp input; duty_b_temp input; duty_c_temp input; duty_b output; duty_c output; duty_a_prev input; duty_b_prev input; duty_c_prev input
function [duty_a,duty_b,duty_c] = fcn(pwm_isr_trig,...
    duty_a_temp,duty_b_temp,duty_c_temp,duty_a_prev,duty_b_prev,duty_c_prev)

if (pwm_isr_trig == 1) % interrupt on prd event
    duty_a = duty_a_temp;
    duty_b = duty_b_temp;
    duty_c = duty_c_temp;
else
    duty_a = duty_a_prev;
    duty_b = duty_b_prev;
    duty_c = duty_c_prev;
end;

== matlab function vbyfcontrolim_interrupt/interrupt generator ==
  data: u1 input; adc_isr_trig output; u2 input; clk input; pwm_isr_trig output; dir output; fsw input; cputimerfreq input; cpu_isr_trig output; start_button input
function [adc_isr_trig,pwm_isr_trig,dir,cpu_isr_trig] = fcn(u1,u2,clk,fsw,...
    cputimerfreq,start_button)

if (rem(clk,1/fsw) == 0)
    adc_isr_trig = 1; % interrupt on zero
    dir = 0;
else
    adc_isr_trig = 0;
    if (u1 > u2)
        dir = 1; % up
    else
        dir = 0; % down
    end;
end;

if (rem(clk*2,1/fsw) == 0 && rem(clk,1/fsw) ~= 0)
    pwm_isr_trig = 1; % interrupt on period
else
    pwm_isr_trig = 0;
end;

if (start_button)
    if (rem(clk,1/cputimerfreq) == 0)
        cpu_isr_trig = 1;
    else
        cpu_isr_trig = 0;
    end
else
    cpu_isr_trig = 0;
end

== matlab function vbyfcontrolim_interrupt/PWM module ==
  data: duty_a input; gate_a1 output; duty_b input; duty_c input; gate_a2 output; gate_b1 output; gate_b2 output; gate_c1 output; gate_c2 output; pwm_counter input; dir input
function [gate_a1,gate_a2,gate_b1,gate_b2,gate_c1,gate_c2] = fcn(duty_a,duty_b,duty_c,pwm_counter,dir)

if (duty_a > pwm_counter)
    gate_a1 = 1;
    gate_a2 = 0;
else
    gate_a1 = 0;
    gate_a2 = 1;
end;
if (duty_b > pwm_counter)
    gate_b1 = 1;
    gate_b2 = 0;
else
    gate_b1 = 0;
    gate_b2 = 1;
end;
if (duty_c > pwm_counter)
    gate_c1 = 1;
    gate_c2 = 0;
else
    gate_c1 = 0;
    gate_c2 = 1;
end;

== matlab function vbyfcontrolim_interrupt/cputimer_isr ==
  data: cpu_isr_trig input; initial_freq input; freq_step input; fsaturation input; Vmax input; start_deceleration input; freq output; ma output; freq_prev input; ma_prev input
function [freq,ma] = fcn(cpu_isr_trig,initial_freq,freq_step,...
    fsaturation,Vmax,start_deceleration,freq_prev,ma_prev)

if (cpu_isr_trig == 1) % interrupt on cputimer event
    if (start_deceleration == 0)
        if (freq_prev + freq_step) > fsaturation
            freq = fsaturation;
        elseif (freq_prev < initial_freq)
            freq = freq_prev + initial_freq;
        else
            freq = freq_prev + freq_step;
        end
    else
        if (freq_prev - freq_step) < 0
            freq = 0;
        else
            freq = freq_prev - freq_step;
        end
    end
    ma = freq*(Vmax/fsaturation)*(sqrt(3)/(750*0.612));
else
    %     if (freq_prev == 0)
    %        freq = initial_freq;
    %     else
    %         freq = freq_prev;
    %     end
    freq = freq_prev;
    ma = ma_prev;
end;
